simulink library "NullAdsbBus"  (R2018b)
settings: Solver=VariableStepAuto  StartTime=0.0  StopTime=10.0  RelTol=1e-3
libraries: signalsLib x1
settings Model: Creator=RA24876  LastModifiedBy=RA24876
settings SFSimCC: SimUseLocalCustomCode=off
settings RTWCC: RTWUseLocalCustomCode=off
settings CodeAppCC: StateflowObjectComments=on

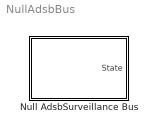
== system NullAdsbBus ==
  Null AdsbSurveillance Bus : Subsystem  mask(Null AdsbSurveillance Bus){}
      mask help: Creates an AdsbSurveillance bus signal with all null values. Assign values to elements with a Bus Assignment block.

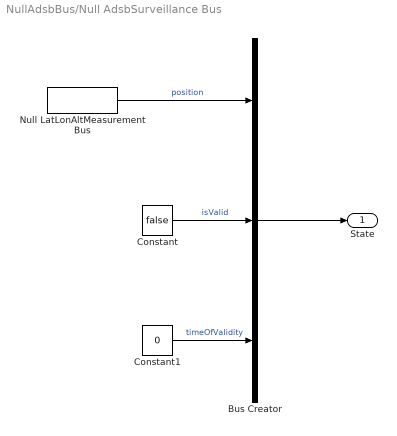
== system NullAdsbBus/Null AdsbSurveillance Bus ==
  Bus Creator : BusCreator  Inputs='latLonAltState','v_ftps','n_ft'  OutDataTypeStr=Bus: AdsbSurveillance
  Constant : Constant  Value=false  OutDataTypeStr=boolean
  Constant1 : Constant  Value=0
  Null LatLonAltMeasurement Bus : signalsLib/Signals/Bus Constructors/Null LatLonAltMeasurement Bus
      settings: SourceProductName=CASSATTv6: Signals Library
  State : Outport  OutDataTypeStr=Bus: AdsbSurveillance
  wires:
  Bus Creator/1 -> State/1
  Constant1/1 -> Bus Creator/3  "timeOfValidity"
  Constant/1 -> Bus Creator/2  "isValid"
  Null LatLonAltMeasurement Bus/1 -> Bus Creator/1  "position"
